simulink model "QueuingSys"  (R2019a)
settings: Solver=VariableStepAuto  StartTime=0.0  StopTime=100  RelTol=1e-3  EnableMultiTasking=on
undefined symbols (not defined in the file or in its folder): m, n
(part 3 of 5)

== system QueuingSys/Distro/MMPPArrivalTime24 ==
  MMPPArrivalTime : TriggerPort  TriggerType=function-call  IsSimulinkFunction=on  FunctionName=MMPPArrivalTime24  VariantControl=Variant
  Constant : Constant  Value=[0.218340938389595 0.112706229136437 0.0913791285356704 0.241717143612315 0.159963629022395 0.101992894543926 0.0739000367596616;0.0360429161526207 0.16434013799063 0.194545292361739 0.260986317842324 0.234076920168349 0.0038388732382826 0.106169542246055;0.140845783996419 0.02142596356304 0.111964255838453 0.214688760468444 0.132405739812884 0.209389328411991 0.169280167908768;0.211603580954734 0.138780880432766 0.228851357631222 0.0929736021625317 0.108365975350849 0.0914026950245187 0.128021908443379;0.196540606477369 0.0424862723550309 0.159462548654797 0.273079768135701 0.0483000474860654 0.264280550522422 0.0158502063686151;0.085539978130616 0.250500965051522 0.0543067416023752 0.49850487643992 0.0486548909117167 0.0235174933555764 0.0389750545082738;0.31220517043653 0.0426377800562429 0.0809275354551289 0.212374582756575 0.0496193007621742 0.129356039135099 0.17287959139825]  SampleTime=-1
  D : Memory  InitialCondition=[0.614629194324132;0.93243288261142]  InheritSampleTime=on
  MMPP : MATLAB Function  TreatAsAtomicUnit=on
  Scope : Scope
  Scope1 : Scope
  T : Memory  InitialCondition=[0 2.63126280993244]  InheritSampleTime=on
  Uniform Random Number : UniformRandomNumber  Minimum=0  Seed=randi(5000)
  X : Memory  InitialCondition=6  InheritSampleTime=on
  t : ArgOut  DisableCoverage=on  ArgumentName=t
  wires:
  MMPP/5(lambda) -> Scope1/1
  D/1 -> MMPP/3("D ")
  MMPP/3(D) -> D/1
  Uniform Random Number/1 -> MMPP/5(rn)
  Constant/1 -> MMPP/4(M)
  MMPP/1(x) -> X/1
  MMPP/4(t) -> Scope/1, t/1
  MMPP/2(T) -> T/1
  T/1 -> MMPP/2("T ")
  X/1 -> MMPP/1("x ")

== system QueuingSys/Distro/MMPPArrivalTime25 ==
  MMPPArrivalTime : TriggerPort  TriggerType=function-call  IsSimulinkFunction=on  FunctionName=MMPPArrivalTime25  VariantControl=Variant
  Constant : Constant  Value=[0.126261776016378 0.256876331205712 0.0743475491381239 0.00987911876596653 0.24041097573006 0.277579906213371 0.0146443429303889;0.215158684388773 0.104699058732068 0.221561488259183 0.114082371425467 0.0931958184132832 0.01898756457891 0.232315014202317;0.14339812125704 0.0963851661286175 0.131725285252208 0.10866184472534 0.104448382274097 0.209437276973192 0.205943923389506;0.11415078083782 0.105394383343145 0.072989249176117 0.0766899189422998 0.184068505318316 0.202592491193927 0.244114671188375;0.280165053993371 0.246511798654403 0.0536757705944194 0.0749268053671436 0.0110419684998257 0.239894108144276 0.0937844947465618;0.127024999749287 0.139114287100631 0.0561443135743664 0.194893192372715 0.202125284585139 0.144969287988396 0.135728634629465;0.0425570718208876 0.00912945422340431 0.179607472937085 0.0477907549956977 0.250445957494757 0.305723190577337 0.16474609795083]  SampleTime=-1
  D : Memory  InitialCondition=[0.84739945723103;0.0464259746177923]  InheritSampleTime=on
  MMPP : MATLAB Function  TreatAsAtomicUnit=on
  Scope : Scope
  Scope1 : Scope
  T : Memory  InitialCondition=[0 0.0425610144779381]  InheritSampleTime=on
  Uniform Random Number : UniformRandomNumber  Minimum=0  Seed=randi(5000)
  X : Memory  InitialCondition=2  InheritSampleTime=on
  t : ArgOut  DisableCoverage=on  ArgumentName=t
  wires:
  MMPP/5(lambda) -> Scope1/1
  D/1 -> MMPP/3("D ")
  MMPP/3(D) -> D/1
  Uniform Random Number/1 -> MMPP/5(rn)
  Constant/1 -> MMPP/4(M)
  MMPP/1(x) -> X/1
  MMPP/4(t) -> Scope/1, t/1
  MMPP/2(T) -> T/1
  T/1 -> MMPP/2("T ")
  X/1 -> MMPP/1("x ")

== system QueuingSys/Distro/MMPPArrivalTime26 ==
  MMPPArrivalTime : TriggerPort  TriggerType=function-call  IsSimulinkFunction=on  FunctionName=MMPPArrivalTime26  VariantControl=Variant
  Constant : Constant  Value=[0.309285239272645 0.083936319045581 0.245188935840708 0.0586916651116355 0.30289784072943;0.249604131350162 0.0262375593681035 0.162014420154344 0.297986672414955 0.264157216712436;0.239496080520532 0.182486674532759 0.050516361065497 0.273833117885605 0.253667765995607;0.323084290176268 0.192126026414458 0.270902867326008 0.0249505358502317 0.188936280233035;0.104368266697699 0.216371091313532 0.330325183296464 0.160531785510462 0.188403673181843]  SampleTime=-1
  D : Memory  InitialCondition=[0.550755647407727;0.0211027090790837]  InheritSampleTime=on
  MMPP : MATLAB Function  TreatAsAtomicUnit=on
  Scope : Scope
  Scope1 : Scope
  T : Memory  InitialCondition=[0 0.0207689449845097]  InheritSampleTime=on
  Uniform Random Number : UniformRandomNumber  Minimum=0  Seed=randi(5000)
  X : Memory  InitialCondition=2  InheritSampleTime=on
  t : ArgOut  DisableCoverage=on  ArgumentName=t
  wires:
  MMPP/5(lambda) -> Scope1/1
  D/1 -> MMPP/3("D ")
  MMPP/3(D) -> D/1
  Uniform Random Number/1 -> MMPP/5(rn)
  Constant/1 -> MMPP/4(M)
  MMPP/1(x) -> X/1
  MMPP/4(t) -> Scope/1, t/1
  MMPP/2(T) -> T/1
  T/1 -> MMPP/2("T ")
  X/1 -> MMPP/1("x ")

== system QueuingSys/Distro/MMPPArrivalTime27 ==
  MMPPArrivalTime : TriggerPort  TriggerType=function-call  IsSimulinkFunction=on  FunctionName=MMPPArrivalTime27  VariantControl=Variant
  Constant : Constant  Value=[0.0196700480561395 0.172600946334506 0.06119529123324 0.251913080143349 0.203718565734216 0.023675877826922 0.267226190671628;0.205861749772008 0.124740430483342 0.0435703487835078 0.259776169203363 0.0251637412405287 0.17177162160965 0.1691159389076;0.0904528149038582 0.0959237307535102 0.0306910128518777 0.237037056690732 0.299086060346327 0.121241544402983 0.125567780050711;0.176070953971679 0.13353863981546 0.0584921398192287 0.131654632433121 0.203364803433442 0.264440012361479 0.0324388181655907;0.00682467460967966 0.136506391709582 0.1695545589303 0.0616100040887452 0.235157640071546 0.244081774115166 0.146264956474981;0.207402505537025 0.0413850634308422 0.182991180389438 0.316311957756415 0.184261630080702 0.0181993774103212 0.0494482853952567;0.145241607470582 0.0447181503479344 0.178772050900297 0.275021549474886 0.104683047120619 0.122449058457546 0.129114536228135]  SampleTime=-1
  D : Memory  InitialCondition=[0.700369541067379;0.242934140773795]  InheritSampleTime=on
  MMPP : MATLAB Function  TreatAsAtomicUnit=on
  Scope : Scope
  Scope1 : Scope
  T : Memory  InitialCondition=[0 0.242371804276988]  InheritSampleTime=on
  Uniform Random Number : UniformRandomNumber  Minimum=0  Seed=randi(5000)
  X : Memory  InitialCondition=7  InheritSampleTime=on
  t : ArgOut  DisableCoverage=on  ArgumentName=t
  wires:
  MMPP/5(lambda) -> Scope1/1
  D/1 -> MMPP/3("D ")
  MMPP/3(D) -> D/1
  Uniform Random Number/1 -> MMPP/5(rn)
  Constant/1 -> MMPP/4(M)
  MMPP/1(x) -> X/1
  MMPP/4(t) -> Scope/1, t/1
  MMPP/2(T) -> T/1
  T/1 -> MMPP/2("T ")
  X/1 -> MMPP/1("x ")

== system QueuingSys/Distro/MMPPArrivalTime28 ==
  MMPPArrivalTime : TriggerPort  TriggerType=function-call  IsSimulinkFunction=on  FunctionName=MMPPArrivalTime28  VariantControl=Variant
  Constant : Constant  Value=[0.1675255939648 0.101797007593022 0.0303730682831272 0.191997428752922 0.177264712643887 0.146387932831963 0.184654255930279;0.0912477542718936 0.210931993970778 0.0843201480116723 0.111897739158023 0.199814913216273 0.20159192162701 0.10019552974435;0.180338394416384 0.0648589650830369 0.154118175392293 0.226715427173359 0.12728298840704 0.0288523571467605 0.217833692381126;0.0172333427169226 0.115598193733394 0.185240713030407 0.185688777825975 0.244050753511532 0.0819293138551697 0.170258905326599;0.157350362929966 0.113879543061761 0.0405457746052219 0.172657753409921 0.145665390816055 0.205649178077014 0.164251997100062;0.0546760945863477 0.153057227941813 0.257667191534973 0.0188514226540526 0.137508337324733 0.175025750837647 0.203213975120434;0.260458682561119 0.122800657363155 0.13819465966866 0.154807542868708 0.145945797704611 0.141207580696075 0.0365850791376733]  SampleTime=-1
  D : Memory  InitialCondition=[0.424539768316478;0.0762116456896338]  InheritSampleTime=on
  MMPP : MATLAB Function  TreatAsAtomicUnit=on
  Scope : Scope
  Scope1 : Scope
  T : Memory  InitialCondition=[0 0.0763721044476675]  InheritSampleTime=on
  Uniform Random Number : UniformRandomNumber  Minimum=0  Seed=randi(5000)
  X : Memory  InitialCondition=7  InheritSampleTime=on
  t : ArgOut  DisableCoverage=on  ArgumentName=t
  wires:
  MMPP/5(lambda) -> Scope1/1
  D/1 -> MMPP/3("D ")
  MMPP/3(D) -> D/1
  Uniform Random Number/1 -> MMPP/5(rn)
  Constant/1 -> MMPP/4(M)
  MMPP/1(x) -> X/1
  MMPP/4(t) -> Scope/1, t/1
  MMPP/2(T) -> T/1
  T/1 -> MMPP/2("T ")
  X/1 -> MMPP/1("x ")

== system QueuingSys/Distro/MMPPArrivalTime29 ==
  MMPPArrivalTime : TriggerPort  TriggerType=function-call  IsSimulinkFunction=on  FunctionName=MMPPArrivalTime29  VariantControl=Variant
  Constant : Constant  Value=[0.470307344262561 0.529692655737439;0.523064675332342 0.476935324667657]  SampleTime=-1
  D : Memory  InitialCondition=[0.726421985150142;0.96965829636015]  InheritSampleTime=on
  MMPP : MATLAB Function  TreatAsAtomicUnit=on
  Scope : Scope
  Scope1 : Scope
  T : Memory  InitialCondition=[0 1.82823247238093]  InheritSampleTime=on
  Uniform Random Number : UniformRandomNumber  Minimum=0  Seed=randi(5000)
  X : Memory  InitialCondition=2  InheritSampleTime=on
  t : ArgOut  DisableCoverage=on  ArgumentName=t
  wires:
  MMPP/5(lambda) -> Scope1/1
  D/1 -> MMPP/3("D ")
  MMPP/3(D) -> D/1
  Uniform Random Number/1 -> MMPP/5(rn)
  Constant/1 -> MMPP/4(M)
  MMPP/1(x) -> X/1
  MMPP/4(t) -> Scope/1, t/1
  MMPP/2(T) -> T/1
  T/1 -> MMPP/2("T ")
  X/1 -> MMPP/1("x ")

== system QueuingSys/Distro/MMPPArrivalTime3 ==
  MMPPArrivalTime : TriggerPort  TriggerType=function-call  IsSimulinkFunction=on  FunctionName=MMPPArrivalTime3  VariantControl=Variant
  Constant : Constant  Value=[0.0853139913388701 0.239102079449207 0.489498373035174 0.186085556176749;0.186029910896899 0.261659421874697 0.139124397204909 0.413186270023495;0.080616426625654 0.578467411552794 0.0755341435246165 0.265382018296936;0.264757301524701 0.239754222585884 0.232748837542538 0.262739638346877]  SampleTime=-1
  D : Memory  InitialCondition=[0.364873259363617;0.592348112171321]  InheritSampleTime=on
  MMPP : MATLAB Function  TreatAsAtomicUnit=on
  Scope : Scope
  Scope1 : Scope
  T : Memory  InitialCondition=[0 0.662543778390372]  InheritSampleTime=on
  Uniform Random Number : UniformRandomNumber  Minimum=0  Seed=randi(5000)
  X : Memory  InitialCondition=2  InheritSampleTime=on
  t : ArgOut  DisableCoverage=on  ArgumentName=t
  wires:
  MMPP/5(lambda) -> Scope1/1
  D/1 -> MMPP/3("D ")
  MMPP/3(D) -> D/1
  Uniform Random Number/1 -> MMPP/5(rn)
  Constant/1 -> MMPP/4(M)
  MMPP/1(x) -> X/1
  MMPP/4(t) -> Scope/1, t/1
  MMPP/2(T) -> T/1
  T/1 -> MMPP/2("T ")
  X/1 -> MMPP/1("x ")

== system QueuingSys/Distro/MMPPArrivalTime30 ==
  MMPPArrivalTime : TriggerPort  TriggerType=function-call  IsSimulinkFunction=on  FunctionName=MMPPArrivalTime30  VariantControl=Variant
  Constant : Constant  Value=[0.206572829547094 0.11219538376502 0.0414783498047576 0.0687166204079749 0.217040951439454 0.0233088998460538 0.330686965189645;0.0588099616266013 0.0794819809807138 0.18046857010927 0.259163205134866 0.1951710016914 0.0924066931854189 0.13449858727173;0.192316426756978 0.190331660158251 0.11812663421486 0.0065555090136078 0.0790712313226722 0.19933171996182 0.214266818571811;0.223545619778498 0.175061907654338 0.150386818941687 0.010317301988908 0.134998537748626 0.173714752944733 0.13197506094321;0.032314357765021 0.23207229786882 0.0750070852278723 0.148072100493113 0.00549085782388581 0.309198074392357 0.197845226428931;0.0617036657326432 0.2510046542784 0.269268599101514 0.0236408275422659 0.0719896733859343 0.318189330143183 0.00420324981605986;0.13091473295952 0.202410050810776 0.0560641524610722 0.212696647631418 0.186442191875069 0.0532754576242078 0.158196766637937]  SampleTime=-1
  D : Memory  InitialCondition=[0.118637485115407;0.596256415905622]  InheritSampleTime=on
  MMPP : MATLAB Function  TreatAsAtomicUnit=on
  Scope : Scope
  Scope1 : Scope
  T : Memory  InitialCondition=[0 0.799837356402608]  InheritSampleTime=on
  Uniform Random Number : UniformRandomNumber  Minimum=0  Seed=randi(5000)
  X : Memory  InitialCondition=3  InheritSampleTime=on
  t : ArgOut  DisableCoverage=on  ArgumentName=t
  wires:
  MMPP/5(lambda) -> Scope1/1
  D/1 -> MMPP/3("D ")
  MMPP/3(D) -> D/1
  Uniform Random Number/1 -> MMPP/5(rn)
  Constant/1 -> MMPP/4(M)
  MMPP/1(x) -> X/1
  MMPP/4(t) -> Scope/1, t/1
  MMPP/2(T) -> T/1
  T/1 -> MMPP/2("T ")
  X/1 -> MMPP/1("x ")

== system QueuingSys/Distro/MMPPArrivalTime31 ==
  MMPPArrivalTime : TriggerPort  TriggerType=function-call  IsSimulinkFunction=on  FunctionName=MMPPArrivalTime31  VariantControl=Variant
  Constant : Constant  Value=[0.551391508708422 0.448608491291578;0.824915716015716 0.175084283984284]  SampleTime=-1
  D : Memory  InitialCondition=[0.92288310288109;0.466638676984603]  InheritSampleTime=on
  MMPP : MATLAB Function  TreatAsAtomicUnit=on
  Scope : Scope
  Scope1 : Scope
  T : Memory  InitialCondition=[0 0.518505871400884]  InheritSampleTime=on
  Uniform Random Number : UniformRandomNumber  Minimum=0  Seed=randi(5000)
  X : Memory  InitialCondition=2  InheritSampleTime=on
  t : ArgOut  DisableCoverage=on  ArgumentName=t
  wires:
  MMPP/5(lambda) -> Scope1/1
  D/1 -> MMPP/3("D ")
  MMPP/3(D) -> D/1
  Uniform Random Number/1 -> MMPP/5(rn)
  Constant/1 -> MMPP/4(M)
  MMPP/1(x) -> X/1
  MMPP/4(t) -> Scope/1, t/1
  MMPP/2(T) -> T/1
  T/1 -> MMPP/2("T ")
  X/1 -> MMPP/1("x ")

== system QueuingSys/Distro/MMPPArrivalTime32 ==
  MMPPArrivalTime : TriggerPort  TriggerType=function-call  IsSimulinkFunction=on  FunctionName=MMPPArrivalTime32  VariantControl=Variant
  Constant : Constant  Value=[0.344522048946834 0.136306917950239 0.243903798161791 0.275267234941136;0.06886895570874 0.352562593749696 0.352121845604469 0.226446604937095;0.30079890177196 0.413635172818291 0.147841511174284 0.137724414235466;0.376216524611495 0.161598610656973 0.00958590106540561 0.452598963666126]  SampleTime=-1
  D : Memory  InitialCondition=[0.488629533539644;0.697627838276884]  InheritSampleTime=on
  MMPP : MATLAB Function  TreatAsAtomicUnit=on
  Scope : Scope
  Scope1 : Scope
  T : Memory  InitialCondition=[0 0.654744571333629]  InheritSampleTime=on
  Uniform Random Number : UniformRandomNumber  Minimum=0  Seed=randi(5000)
  X : Memory  InitialCondition=4  InheritSampleTime=on
  t : ArgOut  DisableCoverage=on  ArgumentName=t
  wires:
  MMPP/5(lambda) -> Scope1/1
  D/1 -> MMPP/3("D ")
  MMPP/3(D) -> D/1
  Uniform Random Number/1 -> MMPP/5(rn)
  Constant/1 -> MMPP/4(M)
  MMPP/1(x) -> X/1
  MMPP/4(t) -> Scope/1, t/1
  MMPP/2(T) -> T/1
  T/1 -> MMPP/2("T ")
  X/1 -> MMPP/1("x ")

== system QueuingSys/Distro/MMPPArrivalTime33 ==
  MMPPArrivalTime : TriggerPort  TriggerType=function-call  IsSimulinkFunction=on  FunctionName=MMPPArrivalTime33  VariantControl=Variant
  Constant : Constant  Value=[0.171570956465584 0.260364817442339 0.320191290579991 0.1239189983333 0.123953937178787;0.179651339948253 0.325383097134665 0.272114117246603 0.0546771683346933 0.168174277335786;0.232175063373843 0.0522707652618958 0.22964458887778 0.278757495659698 0.207152086826784;0.10404887259382 0.143469750206921 0.301159993610954 0.341816203786128 0.109505179802177;0.131507997957578 0.0534805913519804 0.316881075206008 0.419095285263278 0.0790350502211546]  SampleTime=-1
  D : Memory  InitialCondition=[0.347441299611992;0.139538463016827]  InheritSampleTime=on
  MMPP : MATLAB Function  TreatAsAtomicUnit=on
  Scope : Scope
  Scope1 : Scope
  T : Memory  InitialCondition=[0 0.101385720601707]  InheritSampleTime=on
  Uniform Random Number : UniformRandomNumber  Minimum=0  Seed=randi(5000)
  X : Memory  InitialCondition=2  InheritSampleTime=on
  t : ArgOut  DisableCoverage=on  ArgumentName=t
  wires:
  MMPP/5(lambda) -> Scope1/1
  D/1 -> MMPP/3("D ")
  MMPP/3(D) -> D/1
  Uniform Random Number/1 -> MMPP/5(rn)
  Constant/1 -> MMPP/4(M)
  MMPP/1(x) -> X/1
  MMPP/4(t) -> Scope/1, t/1
  MMPP/2(T) -> T/1
  T/1 -> MMPP/2("T ")
  X/1 -> MMPP/1("x ")

== system QueuingSys/Distro/MMPPArrivalTime34 ==
  MMPPArrivalTime : TriggerPort  TriggerType=function-call  IsSimulinkFunction=on  FunctionName=MMPPArrivalTime34  VariantControl=Variant
  Constant : Constant  Value=[0.279863661105788 0.018954509277061 0.701181829617151;0.102024833223184 0.172747068074691 0.725228098702125;0.384615776864446 0.575978320906199 0.0394059022293549]  SampleTime=-1
  D : Memory  InitialCondition=[0.423405961364762;0.537076428867559]  InheritSampleTime=on
  MMPP : MATLAB Function  TreatAsAtomicUnit=on
  Scope : Scope
  Scope1 : Scope
  T : Memory  InitialCondition=[0 0.554644191706879]  InheritSampleTime=on
  Uniform Random Number : UniformRandomNumber  Minimum=0  Seed=randi(5000)
  X : Memory  InitialCondition=1  InheritSampleTime=on
  t : ArgOut  DisableCoverage=on  ArgumentName=t
  wires:
  MMPP/5(lambda) -> Scope1/1
  D/1 -> MMPP/3("D ")
  MMPP/3(D) -> D/1
  Uniform Random Number/1 -> MMPP/5(rn)
  Constant/1 -> MMPP/4(M)
  MMPP/1(x) -> X/1
  MMPP/4(t) -> Scope/1, t/1
  MMPP/2(T) -> T/1
  T/1 -> MMPP/2("T ")
  X/1 -> MMPP/1("x ")

== system QueuingSys/Distro/MMPPArrivalTime35 ==
  MMPPArrivalTime : TriggerPort  TriggerType=function-call  IsSimulinkFunction=on  FunctionName=MMPPArrivalTime35  VariantControl=Variant
  Constant : Constant  Value=[0.188780303843234 0.0823697536250097 0.299442601204683 0.146155756238697 0.283251585088376;0.194799765979573 0.191388575346313 0.213506643310004 0.133027575958572 0.267277439405539;0.16877861121083 0.164421712552048 0.17530282851964 0.169585093051173 0.321911754666309;0.0315952166008945 0.440650528842051 0.356378180470412 0.151542346675446 0.0198337274111962;0.265589533235786 0.370378088201544 0.0329951268661805 0.0974786689921767 0.233558582704313]  SampleTime=-1
  D : Memory  InitialCondition=[0.246188510868016;0.398386263151892]  InheritSampleTime=on
  MMPP : MATLAB Function  TreatAsAtomicUnit=on
  Scope : Scope
  Scope1 : Scope
  T : Memory  InitialCondition=[0 0.419061350834402]  InheritSampleTime=on
  Uniform Random Number : UniformRandomNumber  Minimum=0  Seed=randi(5000)
  X : Memory  InitialCondition=3  InheritSampleTime=on
  t : ArgOut  DisableCoverage=on  ArgumentName=t
  wires:
  MMPP/5(lambda) -> Scope1/1
  D/1 -> MMPP/3("D ")
  MMPP/3(D) -> D/1
  Uniform Random Number/1 -> MMPP/5(rn)
  Constant/1 -> MMPP/4(M)
  MMPP/1(x) -> X/1
  MMPP/4(t) -> Scope/1, t/1
  MMPP/2(T) -> T/1
  T/1 -> MMPP/2("T ")
  X/1 -> MMPP/1("x ")

== system QueuingSys/Distro/MMPPArrivalTime36 ==
  MMPPArrivalTime : TriggerPort  TriggerType=function-call  IsSimulinkFunction=on  FunctionName=MMPPArrivalTime36  VariantControl=Variant
  Constant : Constant  Value=[0.0721368925951376 0.0990877542742027 0.15766762160974 0.173717021931805 0.232520566458114 0.215181743087032 0.0496884000439679;0.104345427832741 0.304945840868097 0.0957926029195893 0.00143421589660746 0.241314256300479 0.00825440376825492 0.243913252414231;0.12349090907902 0.00664393290749279 0.245300465357095 0.0195344479846606 0.147185959478393 0.114720921424828 0.343123363768511;0.0112228226668296 0.212190536597801 0.0609153022626635 0.0522158319742919 0.273310886164233 0.275703567304479 0.114441053029702;0.251806028010796 0.15155975988215 0.0742686826241297 0.0919408199460609 0.0677486819667469 0.324470433888815 0.0382055936813014;0.240353492122863 0.0821997319260256 0.101915103790219 0.153099504996242 0.217093033969166 0.0556167959155748 0.14972233727991;0.203394006302543 0.197611226075048 0.00526531609215853 0.0598232661159766 0.203224493959019 0.165643705328875 0.165037986126379]  SampleTime=-1
  D : Memory  InitialCondition=[0.865261678105272;0.48778428565265]  InheritSampleTime=on
  MMPP : MATLAB Function  TreatAsAtomicUnit=on
  Scope : Scope
  Scope1 : Scope
  T : Memory  InitialCondition=[0 0.620749164508373]  InheritSampleTime=on
  Uniform Random Number : UniformRandomNumber  Minimum=0  Seed=randi(5000)
  X : Memory  InitialCondition=1  InheritSampleTime=on
  t : ArgOut  DisableCoverage=on  ArgumentName=t
  wires:
  MMPP/5(lambda) -> Scope1/1
  D/1 -> MMPP/3("D ")
  MMPP/3(D) -> D/1
  Uniform Random Number/1 -> MMPP/5(rn)
  Constant/1 -> MMPP/4(M)
  MMPP/1(x) -> X/1
  MMPP/4(t) -> Scope/1, t/1
  MMPP/2(T) -> T/1
  T/1 -> MMPP/2("T ")
  X/1 -> MMPP/1("x ")

== system QueuingSys/Distro/MMPPArrivalTime37 ==
  MMPPArrivalTime : TriggerPort  TriggerType=function-call  IsSimulinkFunction=on  FunctionName=MMPPArrivalTime37  VariantControl=Variant
  Constant : Constant  Value=[0.441689750469483 0.131529499484869 0.426780750045648;0.287185036754023 0.0687395784305002 0.644075384815477;0.412359757912282 0.228704386513075 0.358935855574643]  SampleTime=-1
  D : Memory  InitialCondition=[0.206323180349956;0.156967245259197]  InheritSampleTime=on
  MMPP : MATLAB Function  TreatAsAtomicUnit=on
  Scope : Scope
  Scope1 : Scope
  T : Memory  InitialCondition=[0 0.159012220401242]  InheritSampleTime=on
  Uniform Random Number : UniformRandomNumber  Minimum=0  Seed=randi(5000)
  X : Memory  InitialCondition=2  InheritSampleTime=on
  t : ArgOut  DisableCoverage=on  ArgumentName=t
  wires:
  MMPP/5(lambda) -> Scope1/1
  D/1 -> MMPP/3("D ")
  MMPP/3(D) -> D/1
  Uniform Random Number/1 -> MMPP/5(rn)
  Constant/1 -> MMPP/4(M)
  MMPP/1(x) -> X/1
  MMPP/4(t) -> Scope/1, t/1
  MMPP/2(T) -> T/1
  T/1 -> MMPP/2("T ")
  X/1 -> MMPP/1("x ")

== system QueuingSys/Distro/MMPPArrivalTime38 ==
  MMPPArrivalTime : TriggerPort  TriggerType=function-call  IsSimulinkFunction=on  FunctionName=MMPPArrivalTime38  VariantControl=Variant
  Constant : Constant  Value=[0.287926085776875 0.326808914343824 0.140791705619385 0.244473294259917;0.0921151970194848 0.566376965300379 0.244906087745248 0.0966017499348885;0.062348026383559 0.393080925446152 0.351838246969326 0.192732801200964;0.184965879275065 0.287580878998744 0.309163942419966 0.218289299306224]  SampleTime=-1
  D : Memory  InitialCondition=[0.828422805979749;0.99837009190541]  InheritSampleTime=on
  MMPP : MATLAB Function  TreatAsAtomicUnit=on
  Scope : Scope
  Scope1 : Scope
  T : Memory  InitialCondition=[0 4.16070043901108]  InheritSampleTime=on
  Uniform Random Number : UniformRandomNumber  Minimum=0  Seed=randi(5000)
  X : Memory  InitialCondition=3  InheritSampleTime=on
  t : ArgOut  DisableCoverage=on  ArgumentName=t
  wires:
  MMPP/5(lambda) -> Scope1/1
  D/1 -> MMPP/3("D ")
  MMPP/3(D) -> D/1
  Uniform Random Number/1 -> MMPP/5(rn)
  Constant/1 -> MMPP/4(M)
  MMPP/1(x) -> X/1
  MMPP/4(t) -> Scope/1, t/1
  MMPP/2(T) -> T/1
  T/1 -> MMPP/2("T ")
  X/1 -> MMPP/1("x ")

== system QueuingSys/Distro/MMPPArrivalTime39 ==
  MMPPArrivalTime : TriggerPort  TriggerType=function-call  IsSimulinkFunction=on  FunctionName=MMPPArrivalTime39  VariantControl=Variant
  Constant : Constant  Value=[0.203369723433177 0.0981529295965351 0.27974031168011 0.418737035290178;0.118401652360432 0.343942875686384 0.483441151549918 0.0542143204032651;0.57842810044429 0.0186327882062443 0.0993934778872626 0.303545633462203;0.181636059897378 0.250261790687725 0.21359752945179 0.354504619963107]  SampleTime=-1
  D : Memory  InitialCondition=[0.700194935136202;0.830731114447627]  InheritSampleTime=on
  MMPP : MATLAB Function  TreatAsAtomicUnit=on
  Scope : Scope
  Scope1 : Scope
  T : Memory  InitialCondition=[0 1.41502790389446]  InheritSampleTime=on
  Uniform Random Number : UniformRandomNumber  Minimum=0  Seed=randi(5000)
  X : Memory  InitialCondition=1  InheritSampleTime=on
  t : ArgOut  DisableCoverage=on  ArgumentName=t
  wires:
  MMPP/5(lambda) -> Scope1/1
  D/1 -> MMPP/3("D ")
  MMPP/3(D) -> D/1
  Uniform Random Number/1 -> MMPP/5(rn)
  Constant/1 -> MMPP/4(M)
  MMPP/1(x) -> X/1
  MMPP/4(t) -> Scope/1, t/1
  MMPP/2(T) -> T/1
  T/1 -> MMPP/2("T ")
  X/1 -> MMPP/1("x ")

== system QueuingSys/Distro/MMPPArrivalTime4 ==
  MMPPArrivalTime : TriggerPort  TriggerType=function-call  IsSimulinkFunction=on  FunctionName=MMPPArrivalTime4  VariantControl=Variant
  Constant : Constant  Value=[0.0222433821916003 0.188004075907925 0.0437472879804383 0.12935035710123 0.178735535005156 0.182042759176272 0.0734492807049325 0.182427321932446;0.114137403815038 0.118952869883947 0.173447243215089 0.0309547927779365 0.09532864645341 0.142509570506958 0.0965657578792342 0.228103715468389;0.149811893306025 0.0250072529977261 0.082539304657149 0.106939407254426 0.184206355648754 0.186347503583938 0.0910378188644563 0.174110463687526;0.199110919696702 0.0774059631971286 0.114567260154314 0.166430806338449 0.0700866595008907 0.191021231764798 0.154458031307493 0.0269191280402247;0.136518653768493 0.189298811903415 0.0490924625299025 0.0850191815014507 0.113079738549474 0.0120577465523648 0.226651515000193 0.188281890194708;0.010143876364335 0.212656924819349 0.0912173901823647 0.115440804587796 0.0551317551617981 0.226660862641394 0.14582232951616 0.142926056726803;0.129649913543163 0.154270484050175 0.0757750971600601 0.0262850321230364 0.171745147765562 0.140824816060237 0.212889797246578 0.088559712051188;0.0675108333403751 0.235392828283239 0.0864519004234807 0.139572546540988 0.06630522993186 0.0176149303934803 0.183129017966379 0.204022713120198]  SampleTime=-1
  D : Memory  InitialCondition=[0.0962059280401967;0.948102236245469]  InheritSampleTime=on
  MMPP : MATLAB Function  TreatAsAtomicUnit=on
  Scope : Scope
  Scope1 : Scope
  T : Memory  InitialCondition=[0 2.89267298537551]  InheritSampleTime=on
  Uniform Random Number : UniformRandomNumber  Minimum=0  Seed=randi(5000)
  X : Memory  InitialCondition=1  InheritSampleTime=on
  t : ArgOut  DisableCoverage=on  ArgumentName=t
  wires:
  MMPP/5(lambda) -> Scope1/1
  D/1 -> MMPP/3("D ")
  MMPP/3(D) -> D/1
  Uniform Random Number/1 -> MMPP/5(rn)
  Constant/1 -> MMPP/4(M)
  MMPP/1(x) -> X/1
  MMPP/4(t) -> Scope/1, t/1
  MMPP/2(T) -> T/1
  T/1 -> MMPP/2("T ")
  X/1 -> MMPP/1("x ")

== system QueuingSys/Distro/MMPPArrivalTime40 ==
  MMPPArrivalTime : TriggerPort  TriggerType=function-call  IsSimulinkFunction=on  FunctionName=MMPPArrivalTime40  VariantControl=Variant
  Constant : Constant  Value=[0.307578865869595 0.132038010112806 0.121090750876633 0.221383495684156 0.21790887745681;0.0744758422654912 0.243685342092243 0.270264233257038 0.242878524139999 0.16869605824523;0.0720937486394534 0.228376662965373 0.214644675250443 0.235434871797632 0.249450041347098;0.213128802454875 0.258371791749583 0.259796810506448 0.00747698392181957 0.261225611367275;0.231301535709266 0.178744002603726 0.184654760537249 0.173233407727554 0.232066293422205]  SampleTime=-1
  D : Memory  InitialCondition=[0.277363250387578;0.316407242248477]  InheritSampleTime=on
  MMPP : MATLAB Function  TreatAsAtomicUnit=on
  Scope : Scope
  Scope1 : Scope
  T : Memory  InitialCondition=[0 0.287696742729591]  InheritSampleTime=on
  Uniform Random Number : UniformRandomNumber  Minimum=0  Seed=randi(5000)
  X : Memory  InitialCondition=2  InheritSampleTime=on
  t : ArgOut  DisableCoverage=on  ArgumentName=t
  wires:
  MMPP/5(lambda) -> Scope1/1
  D/1 -> MMPP/3("D ")
  MMPP/3(D) -> D/1
  Uniform Random Number/1 -> MMPP/5(rn)
  Constant/1 -> MMPP/4(M)
  MMPP/1(x) -> X/1
  MMPP/4(t) -> Scope/1, t/1
  MMPP/2(T) -> T/1
  T/1 -> MMPP/2("T ")
  X/1 -> MMPP/1("x ")

== system QueuingSys/Distro/MMPPArrivalTime41 ==
  MMPPArrivalTime : TriggerPort  TriggerType=function-call  IsSimulinkFunction=on  FunctionName=MMPPArrivalTime41  VariantControl=Variant
  Constant : Constant  Value=[0.410876353322907 0.0584260983388013 0.337581915528107 0.193115632810185;0.335369397531136 0.236701922750816 0.19284870942629 0.235079970291758;0.202496633153807 0.0925488926150038 0.323559931884597 0.381394542346592;0.232535225417897 0.0796771501394147 0.072060247438763 0.615727377003925]  SampleTime=-1
  D : Memory  InitialCondition=[0.372362436968764;0.102235461961869]  InheritSampleTime=on
  MMPP : MATLAB Function  TreatAsAtomicUnit=on
  Scope : Scope
  Scope1 : Scope
  T : Memory  InitialCondition=[0 0.0823197528598087]  InheritSampleTime=on
  Uniform Random Number : UniformRandomNumber  Minimum=0  Seed=randi(5000)
  X : Memory  InitialCondition=2  InheritSampleTime=on
  t : ArgOut  DisableCoverage=on  ArgumentName=t
  wires:
  MMPP/5(lambda) -> Scope1/1
  D/1 -> MMPP/3("D ")
  MMPP/3(D) -> D/1
  Uniform Random Number/1 -> MMPP/5(rn)
  Constant/1 -> MMPP/4(M)
  MMPP/1(x) -> X/1
  MMPP/4(t) -> Scope/1, t/1
  MMPP/2(T) -> T/1
  T/1 -> MMPP/2("T ")
  X/1 -> MMPP/1("x ")

== system QueuingSys/Distro/MMPPArrivalTime42 ==
  MMPPArrivalTime : TriggerPort  TriggerType=function-call  IsSimulinkFunction=on  FunctionName=MMPPArrivalTime42  VariantControl=Variant
  Constant : Constant  Value=[0.19484043500199 0.284944522797008 0.0475706332073199 0.109134773917783 0.239436419068973 0.124073216006926;0.126050594916668 0.261824844654131 0.0248899095858524 0.311802037053651 0.215696750369367 0.0597358634203302;0.0495412974773776 0.210291104549826 0.16361300927134 0.279547564424455 0.191625022747464 0.105382001529537;0.154861130114456 0.239858888632055 0.0256755968521409 0.261586392968357 0.0592600681071114 0.25875792332588;0.244180818964456 0.22217501763753 0.1126239642831 0.0654110364937203 0.137653601903044 0.217955560718149;0.400637514695211 0.318208115296665 0.130290915360653 0.0202519126212345 0.0232855982319286 0.107325943794308]  SampleTime=-1
  D : Memory  InitialCondition=[0.733514334816772;0.782224136821224]  InheritSampleTime=on
  MMPP : MATLAB Function  TreatAsAtomicUnit=on
  Scope : Scope
  Scope1 : Scope
  T : Memory  InitialCondition=[0 1.2748954024409]  InheritSampleTime=on
  Uniform Random Number : UniformRandomNumber  Minimum=0  Seed=randi(5000)
  X : Memory  InitialCondition=3  InheritSampleTime=on
  t : ArgOut  DisableCoverage=on  ArgumentName=t
  wires:
  MMPP/5(lambda) -> Scope1/1
  D/1 -> MMPP/3("D ")
  MMPP/3(D) -> D/1
  Uniform Random Number/1 -> MMPP/5(rn)
  Constant/1 -> MMPP/4(M)
  MMPP/1(x) -> X/1
  MMPP/4(t) -> Scope/1, t/1
  MMPP/2(T) -> T/1
  T/1 -> MMPP/2("T ")
  X/1 -> MMPP/1("x ")

== system QueuingSys/Distro/MMPPArrivalTime43 ==
  MMPPArrivalTime : TriggerPort  TriggerType=function-call  IsSimulinkFunction=on  FunctionName=MMPPArrivalTime43  VariantControl=Variant
  Constant : Constant  Value=[0.666230645010512 0.333769354989488;0.648952377526222 0.351047622473778]  SampleTime=-1
  D : Memory  InitialCondition=[0.695748329396229;0.694899405806817]  InheritSampleTime=on
  MMPP : MATLAB Function  TreatAsAtomicUnit=on
  Scope : Scope
  Scope1 : Scope
  T : Memory  InitialCondition=[0 0.770380283788956]  InheritSampleTime=on
  Uniform Random Number : UniformRandomNumber  Minimum=0  Seed=randi(5000)
  X : Memory  InitialCondition=2  InheritSampleTime=on
  t : ArgOut  DisableCoverage=on  ArgumentName=t
  wires:
  MMPP/5(lambda) -> Scope1/1
  D/1 -> MMPP/3("D ")
  MMPP/3(D) -> D/1
  Uniform Random Number/1 -> MMPP/5(rn)
  Constant/1 -> MMPP/4(M)
  MMPP/1(x) -> X/1
  MMPP/4(t) -> Scope/1, t/1
  MMPP/2(T) -> T/1
  T/1 -> MMPP/2("T ")
  X/1 -> MMPP/1("x ")

== system QueuingSys/Distro/MMPPArrivalTime44 ==
  MMPPArrivalTime : TriggerPort  TriggerType=function-call  IsSimulinkFunction=on  FunctionName=MMPPArrivalTime44  VariantControl=Variant
  Constant : Constant  Value=[0.15203561034492 0.187503181484866 0.217099640527759 0.261940593187943 0.111892281007731 0.000650429792438285 0.0688782636543432;0.0629211458311256 0.261964703771416 0.195749518075014 0.0286599345113848 0.245131323254798 0.102903898094534 0.102669476461728;0.200682855577231 0.138658530834025 0.143251811474266 0.0529877333897891 0.138171464438406 0.141119359774842 0.18512824451144;0.191890770111757 0.437124293431787 0.0315258938631034 0.226728507658625 0.0913806175234772 0.0203987673434622 0.000951150067788178;0.136393955971383 0.0241916835568405 0.18780202494869 0.163005280150987 0.179085451974293 0.120692281793856 0.188829321603951;0.148892943828847 0.235368435604696 0.170914905612149 0.170876773227261 0.0196435783696241 0.0970585690252984 0.157244794332124;0.160582990055915 0.0115380956607863 0.0970534935676632 0.121345310071338 0.21807668732859 0.162514380533904 0.228889042781804]  SampleTime=-1
  D : Memory  InitialCondition=[0.390100290285044;0.951080809713353]  InheritSampleTime=on
  MMPP : MATLAB Function  TreatAsAtomicUnit=on
  Scope : Scope
  Scope1 : Scope
  T : Memory  InitialCondition=[0 2.58531092805497]  InheritSampleTime=on
  Uniform Random Number : UniformRandomNumber  Minimum=0  Seed=randi(5000)
  X : Memory  InitialCondition=3  InheritSampleTime=on
  t : ArgOut  DisableCoverage=on  ArgumentName=t
  wires:
  MMPP/5(lambda) -> Scope1/1
  D/1 -> MMPP/3("D ")
  MMPP/3(D) -> D/1
  Uniform Random Number/1 -> MMPP/5(rn)
  Constant/1 -> MMPP/4(M)
  MMPP/1(x) -> X/1
  MMPP/4(t) -> Scope/1, t/1
  MMPP/2(T) -> T/1
  T/1 -> MMPP/2("T ")
  X/1 -> MMPP/1("x ")

== system QueuingSys/Distro/MMPPArrivalTime45 ==
  MMPPArrivalTime : TriggerPort  TriggerType=function-call  IsSimulinkFunction=on  FunctionName=MMPPArrivalTime45  VariantControl=Variant
  Constant : Constant  Value=[0.208332003253337 0.0984433340257894 0.0275476333176013 0.208455019743088 0.187769647373873 0.138168787674138 0.131283574612174;0.119543919326924 0.030488950877573 0.176370764184541 0.179747392102269 0.16774180681458 0.183564418114314 0.142542748579799;0.0172780841585348 0.295546396625372 0.258578259992568 0.227118085955286 0.132218391124284 0.0520412705413815 0.0172195116025731;0.351815240726735 0.0479964117693768 0.0570504295879172 0.233496406215703 0.0264590985001854 0.265698725665895 0.0174836875341881;0.0156438106290037 0.203879845806784 0.106041292079691 0.227281290089628 0.244940838010454 0.0449931946230161 0.157219728761424;0.078251026730738 0.201058916592686 0.145343733254437 0.118734781147526 0.192447945467668 0.0249161137048323 0.239247483102113;0.0964831958453108 0.0788638465842378 0.189772507959354 0.231147832892259 0.192992728438768 0.163089502009768 0.0476503862703027]  SampleTime=-1
  D : Memory  InitialCondition=[0.573696348603338;0.604938867660859]  InheritSampleTime=on
  MMPP : MATLAB Function  TreatAsAtomicUnit=on
  Scope : Scope
  Scope1 : Scope
  T : Memory  InitialCondition=[0 0.71186320163139]  InheritSampleTime=on
  Uniform Random Number : UniformRandomNumber  Minimum=0  Seed=randi(5000)
  X : Memory  InitialCondition=4  InheritSampleTime=on
  t : ArgOut  DisableCoverage=on  ArgumentName=t
  wires:
  MMPP/5(lambda) -> Scope1/1
  D/1 -> MMPP/3("D ")
  MMPP/3(D) -> D/1
  Uniform Random Number/1 -> MMPP/5(rn)
  Constant/1 -> MMPP/4(M)
  MMPP/1(x) -> X/1
  MMPP/4(t) -> Scope/1, t/1
  MMPP/2(T) -> T/1
  T/1 -> MMPP/2("T ")
  X/1 -> MMPP/1("x ")

== system QueuingSys/Distro/MMPPArrivalTime46 ==
  MMPPArrivalTime : TriggerPort  TriggerType=function-call  IsSimulinkFunction=on  FunctionName=MMPPArrivalTime46  VariantControl=Variant
  Constant : Constant  Value=[0.526814867969532 0.473185132030468;0.0348504552695229 0.965149544730477]  SampleTime=-1
  D : Memory  InitialCondition=[0.370318725663683;0.075636685022303]  InheritSampleTime=on
  MMPP : MATLAB Function  TreatAsAtomicUnit=on
  Scope : Scope
  Scope1 : Scope
  T : Memory  InitialCondition=[0 0.0372160516095348]  InheritSampleTime=on
  Uniform Random Number : UniformRandomNumber  Minimum=0  Seed=randi(5000)
  X : Memory  InitialCondition=1  InheritSampleTime=on
  t : ArgOut  DisableCoverage=on  ArgumentName=t
  wires:
  MMPP/5(lambda) -> Scope1/1
  D/1 -> MMPP/3("D ")
  MMPP/3(D) -> D/1
  Uniform Random Number/1 -> MMPP/5(rn)
  Constant/1 -> MMPP/4(M)
  MMPP/1(x) -> X/1
  MMPP/4(t) -> Scope/1, t/1
  MMPP/2(T) -> T/1
  T/1 -> MMPP/2("T ")
  X/1 -> MMPP/1("x ")

== system QueuingSys/Distro/MMPPArrivalTime47 ==
  MMPPArrivalTime : TriggerPort  TriggerType=function-call  IsSimulinkFunction=on  FunctionName=MMPPArrivalTime47  VariantControl=Variant
  Constant : Constant  Value=[0.357649279094256 0.383062766136625 0.259287954769119;0.18487698933807 0.307582643317699 0.507540367344231;0.302376740201481 0.447645097081492 0.249978162717027]  SampleTime=-1
  D : Memory  InitialCondition=[0.929496207556362;0.418572454279479]  InheritSampleTime=on
  MMPP : MATLAB Function  TreatAsAtomicUnit=on
  Scope : Scope
  Scope1 : Scope
  T : Memory  InitialCondition=[0 0.348326827652435]  InheritSampleTime=on
  Uniform Random Number : UniformRandomNumber  Minimum=0  Seed=randi(5000)
  X : Memory  InitialCondition=1  InheritSampleTime=on
  t : ArgOut  DisableCoverage=on  ArgumentName=t
  wires:
  MMPP/5(lambda) -> Scope1/1
  D/1 -> MMPP/3("D ")
  MMPP/3(D) -> D/1
  Uniform Random Number/1 -> MMPP/5(rn)
  Constant/1 -> MMPP/4(M)
  MMPP/1(x) -> X/1
  MMPP/4(t) -> Scope/1, t/1
  MMPP/2(T) -> T/1
  T/1 -> MMPP/2("T ")
  X/1 -> MMPP/1("x ")

== system QueuingSys/Distro/MMPPArrivalTime48 ==
  MMPPArrivalTime : TriggerPort  TriggerType=function-call  IsSimulinkFunction=on  FunctionName=MMPPArrivalTime48  VariantControl=Variant
  Constant : Constant  Value=[0.0989361828816905 0.178257670888535 0.142181889481987 0.322312499159869 0.258311757587918;0.225531062681923 0.243602356421045 0.15415192697207 0.165161105172416 0.211553548752546;0.205474509467409 0.190905839449352 0.183780085282627 0.165890917526993 0.253948648273619;0.346999335019431 0.174541386602823 0.0398510890529728 0.0705196289089337 0.36808856041584;0.167273984423134 0.205900307853727 0.113969465774524 0.108299928616902 0.404556313331712]  SampleTime=-1
  D : Memory  InitialCondition=[0.529638235684598;0.288370830577306]  InheritSampleTime=on
  MMPP : MATLAB Function  TreatAsAtomicUnit=on
  Scope : Scope
  Scope1 : Scope
  T : Memory  InitialCondition=[0 0.202568949428109]  InheritSampleTime=on
  Uniform Random Number : UniformRandomNumber  Minimum=0  Seed=randi(5000)
  X : Memory  InitialCondition=5  InheritSampleTime=on
  t : ArgOut  DisableCoverage=on  ArgumentName=t
  wires:
  MMPP/5(lambda) -> Scope1/1
  D/1 -> MMPP/3("D ")
  MMPP/3(D) -> D/1
  Uniform Random Number/1 -> MMPP/5(rn)
  Constant/1 -> MMPP/4(M)
  MMPP/1(x) -> X/1
  MMPP/4(t) -> Scope/1, t/1
  MMPP/2(T) -> T/1
  T/1 -> MMPP/2("T ")
  X/1 -> MMPP/1("x ")

== system QueuingSys/Distro/MMPPArrivalTime49 ==
  MMPPArrivalTime : TriggerPort  TriggerType=function-call  IsSimulinkFunction=on  FunctionName=MMPPArrivalTime49  VariantControl=Variant
  Constant : Constant  Value=[0.0169370390093233 0.573595038383496 0.409467922607181;0.279966128744602 0.301329869356476 0.418704001898922;0.00372472863765805 0.113664329342455 0.882610942019887]  SampleTime=-1
  D : Memory  InitialCondition=[0.523322004017897;0.392486014299919]  InheritSampleTime=on
  MMPP : MATLAB Function  TreatAsAtomicUnit=on
  Scope : Scope
  Scope1 : Scope
  T : Memory  InitialCondition=[0 0.348203277213396]  InheritSampleTime=on
  Uniform Random Number : UniformRandomNumber  Minimum=0  Seed=randi(5000)
  X : Memory  InitialCondition=2  InheritSampleTime=on
  t : ArgOut  DisableCoverage=on  ArgumentName=t
  wires:
  MMPP/5(lambda) -> Scope1/1
  D/1 -> MMPP/3("D ")
  MMPP/3(D) -> D/1
  Uniform Random Number/1 -> MMPP/5(rn)
  Constant/1 -> MMPP/4(M)
  MMPP/1(x) -> X/1
  MMPP/4(t) -> Scope/1, t/1
  MMPP/2(T) -> T/1
  T/1 -> MMPP/2("T ")
  X/1 -> MMPP/1("x ")

== system QueuingSys/Distro/MMPPArrivalTime5 ==
  MMPPArrivalTime : TriggerPort  TriggerType=function-call  IsSimulinkFunction=on  FunctionName=MMPPArrivalTime5  VariantControl=Variant
  Constant : Constant  Value=[0.190433648778553 0.311290627479789 0.290257210078387 0.208018513663271;0.0545287179524431 0.45550681599807 0.213399191698696 0.276565274350791;0.32709725875407 0.0520384576738759 0.247760062991669 0.373104220580386;0.321656492085376 0.499520802863322 0.0497368589714937 0.129085846079808]  SampleTime=-1
  D : Memory  InitialCondition=[0.193494994981051;0.53092770419017]  InheritSampleTime=on
  MMPP : MATLAB Function  TreatAsAtomicUnit=on
  Scope : Scope
  Scope1 : Scope
  T : Memory  InitialCondition=[0 0.659280598034344]  InheritSampleTime=on
  Uniform Random Number : UniformRandomNumber  Minimum=0  Seed=randi(5000)
  X : Memory  InitialCondition=4  InheritSampleTime=on
  t : ArgOut  DisableCoverage=on  ArgumentName=t
  wires:
  MMPP/5(lambda) -> Scope1/1
  D/1 -> MMPP/3("D ")
  MMPP/3(D) -> D/1
  Uniform Random Number/1 -> MMPP/5(rn)
  Constant/1 -> MMPP/4(M)
  MMPP/1(x) -> X/1
  MMPP/4(t) -> Scope/1, t/1
  MMPP/2(T) -> T/1
  T/1 -> MMPP/2("T ")
  X/1 -> MMPP/1("x ")

== system QueuingSys/Distro/MMPPArrivalTime50 ==
  MMPPArrivalTime : TriggerPort  TriggerType=function-call  IsSimulinkFunction=on  FunctionName=MMPPArrivalTime50  VariantControl=Variant
  Constant : Constant  Value=[0.710640218684484 0.289359781315516;0.438035940675537 0.561964059324463]  SampleTime=-1
  D : Memory  InitialCondition=[0.737876332989012;0.13841777189992]  InheritSampleTime=on
  MMPP : MATLAB Function  TreatAsAtomicUnit=on
  Scope : Scope
  Scope1 : Scope
  T : Memory  InitialCondition=[0 0.065260688243774]  InheritSampleTime=on
  Uniform Random Number : UniformRandomNumber  Minimum=0  Seed=randi(5000)
  X : Memory  InitialCondition=2  InheritSampleTime=on
  t : ArgOut  DisableCoverage=on  ArgumentName=t
  wires:
  MMPP/5(lambda) -> Scope1/1
  D/1 -> MMPP/3("D ")
  MMPP/3(D) -> D/1
  Uniform Random Number/1 -> MMPP/5(rn)
  Constant/1 -> MMPP/4(M)
  MMPP/1(x) -> X/1
  MMPP/4(t) -> Scope/1, t/1
  MMPP/2(T) -> T/1
  T/1 -> MMPP/2("T ")
  X/1 -> MMPP/1("x ")

== system QueuingSys/Distro/MMPPArrivalTime51 ==
  MMPPArrivalTime : TriggerPort  TriggerType=function-call  IsSimulinkFunction=on  FunctionName=MMPPArrivalTime51  VariantControl=Variant
  Constant : Constant  Value=[0.27477589633085 0.72522410366915;0.576167588252239 0.423832411747761]  SampleTime=-1
  D : Memory  InitialCondition=[0.679664293958122;0.0795688618013785]  InheritSampleTime=on
  MMPP : MATLAB Function  TreatAsAtomicUnit=on
  Scope : Scope
  Scope1 : Scope
  T : Memory  InitialCondition=[0 0.0601305715476238]  InheritSampleTime=on
  Uniform Random Number : UniformRandomNumber  Minimum=0  Seed=randi(5000)
  X : Memory  InitialCondition=1  InheritSampleTime=on
  t : ArgOut  DisableCoverage=on  ArgumentName=t
  wires:
  MMPP/5(lambda) -> Scope1/1
  D/1 -> MMPP/3("D ")
  MMPP/3(D) -> D/1
  Uniform Random Number/1 -> MMPP/5(rn)
  Constant/1 -> MMPP/4(M)
  MMPP/1(x) -> X/1
  MMPP/4(t) -> Scope/1, t/1
  MMPP/2(T) -> T/1
  T/1 -> MMPP/2("T ")
  X/1 -> MMPP/1("x ")

== system QueuingSys/Distro/MMPPArrivalTime52 ==
  MMPPArrivalTime : TriggerPort  TriggerType=function-call  IsSimulinkFunction=on  FunctionName=MMPPArrivalTime52  VariantControl=Variant
  Constant : Constant  Value=[0.0779456373812396 0.225274098754333 0.135235329503905 0.322160116791718 0.239384817568805;0.237603595831951 0.195901606332091 0.209668820848791 0.117585415067075 0.239240561920092;0.10094128161487 0.306255810576098 0.105545511079908 0.235267858982242 0.251989537746883;0.0317906697226869 0.0912138240831371 0.361158339860435 0.418438011318553 0.0973991550151886;0.344674187629098 0.328778261982713 0.177310589680979 0.0983342844648327 0.050902676242377]  SampleTime=-1
  D : Memory  InitialCondition=[0.980096005521268;0.751684027310974]  InheritSampleTime=on
  MMPP : MATLAB Function  TreatAsAtomicUnit=on
  Scope : Scope
  Scope1 : Scope
  T : Memory  InitialCondition=[0 1.32214312124926]  InheritSampleTime=on
  Uniform Random Number : UniformRandomNumber  Minimum=0  Seed=randi(5000)
  X : Memory  InitialCondition=5  InheritSampleTime=on
  t : ArgOut  DisableCoverage=on  ArgumentName=t
  wires:
  MMPP/5(lambda) -> Scope1/1
  D/1 -> MMPP/3("D ")
  MMPP/3(D) -> D/1
  Uniform Random Number/1 -> MMPP/5(rn)
  Constant/1 -> MMPP/4(M)
  MMPP/1(x) -> X/1
  MMPP/4(t) -> Scope/1, t/1
  MMPP/2(T) -> T/1
  T/1 -> MMPP/2("T ")
  X/1 -> MMPP/1("x ")

== system QueuingSys/Distro/MMPPArrivalTime53 ==
  MMPPArrivalTime : TriggerPort  TriggerType=function-call  IsSimulinkFunction=on  FunctionName=MMPPArrivalTime53  VariantControl=Variant
  Constant : Constant  Value=[0.123213782072751 0.0203564984206003 0.257051566111025 0.0145943311681688 0.0816876671703166 0.134023465595343 0.2585969637835 0.110475725678296;0.0177158527683463 0.194973002202457 0.12651531765153 0.114307978366439 0.0161070662064469 0.155504816989333 0.161669538323955 0.213206427491493;0.0344595627708055 0.124382621870903 0.173362716325991 0.0550418448821959 0.182709438022144 0.166633381790352 0.093981667089674 0.169428767247933;0.170175469423192 0.0369170999924753 0.013784091076386 0.147927274138185 0.0958134249132087 0.195744315289456 0.19364534372614 0.145992981440957;0.201811926034737 0.11150230943796 0.14620939075993 0.132613560755162 0.168392899815457 0.18383901638292 0.0311142203307919 0.024516676483042;0.185902766042658 0.153371383875054 0.0286654140386129 0.0177500774355355 0.266231807527502 0.0101540434889089 0.189511404901813 0.148413102689917;0.0941915976279465 0.113587544400254 0.11079634693523 0.162219066048839 0.158751736041027 0.164944426900267 0.107942998113772 0.0875662839326654;0.125359025190266 0.172346379619826 0.143719398120004 0.170339054795389 0.172131272820563 0.112197209524467 0.0917269017918102 0.0121807581376756]  SampleTime=-1
  D : Memory  InitialCondition=[0.805203215911553;0.786655637028361]  InheritSampleTime=on
  MMPP : MATLAB Function  TreatAsAtomicUnit=on
  Scope : Scope
  Scope1 : Scope
  T : Memory  InitialCondition=[0 1.31632258328505]  InheritSampleTime=on
  Uniform Random Number : UniformRandomNumber  Minimum=0  Seed=randi(5000)
  X : Memory  InitialCondition=4  InheritSampleTime=on
  t : ArgOut  DisableCoverage=on  ArgumentName=t
  wires:
  MMPP/5(lambda) -> Scope1/1
  D/1 -> MMPP/3("D ")
  MMPP/3(D) -> D/1
  Uniform Random Number/1 -> MMPP/5(rn)
  Constant/1 -> MMPP/4(M)
  MMPP/1(x) -> X/1
  MMPP/4(t) -> Scope/1, t/1
  MMPP/2(T) -> T/1
  T/1 -> MMPP/2("T ")
  X/1 -> MMPP/1("x ")

== system QueuingSys/Distro/MMPPArrivalTime54 ==
  MMPPArrivalTime : TriggerPort  TriggerType=function-call  IsSimulinkFunction=on  FunctionName=MMPPArrivalTime54  VariantControl=Variant
  Constant : Constant  Value=[0.0425375316354311 0.957462468364569;0.493384015353972 0.506615984646028]  SampleTime=-1
  D : Memory  InitialCondition=[0.48914740808751;0.284127022809931]  InheritSampleTime=on
  MMPP : MATLAB Function  TreatAsAtomicUnit=on
  Scope : Scope
  Scope1 : Scope
  T : Memory  InitialCondition=[0 0.320034256183147]  InheritSampleTime=on
  Uniform Random Number : UniformRandomNumber  Minimum=0  Seed=randi(5000)
  X : Memory  InitialCondition=1  InheritSampleTime=on
  t : ArgOut  DisableCoverage=on  ArgumentName=t
  wires:
  MMPP/5(lambda) -> Scope1/1
  D/1 -> MMPP/3("D ")
  MMPP/3(D) -> D/1
  Uniform Random Number/1 -> MMPP/5(rn)
  Constant/1 -> MMPP/4(M)
  MMPP/1(x) -> X/1
  MMPP/4(t) -> Scope/1, t/1
  MMPP/2(T) -> T/1
  T/1 -> MMPP/2("T ")
  X/1 -> MMPP/1("x ")

== system QueuingSys/Distro/MMPPArrivalTime55 ==
  MMPPArrivalTime : TriggerPort  TriggerType=function-call  IsSimulinkFunction=on  FunctionName=MMPPArrivalTime55  VariantControl=Variant
  Constant : Constant  Value=[0.322744310179396 0.161126721845851 0.516128967974753;0.393346289404341 0.250659781843798 0.35599392875186;0.360441015160688 0.329883638020048 0.309675346819264]  SampleTime=-1
  D : Memory  InitialCondition=[0.355807120256821;0.193194442421816]  InheritSampleTime=on
  MMPP : MATLAB Function  TreatAsAtomicUnit=on
  Scope : Scope
  Scope1 : Scope
  T : Memory  InitialCondition=[0 0.148193777445589]  InheritSampleTime=on
  Uniform Random Number : UniformRandomNumber  Minimum=0  Seed=randi(5000)
  X : Memory  InitialCondition=3  InheritSampleTime=on
  t : ArgOut  DisableCoverage=on  ArgumentName=t
  wires:
  MMPP/5(lambda) -> Scope1/1
  D/1 -> MMPP/3("D ")
  MMPP/3(D) -> D/1
  Uniform Random Number/1 -> MMPP/5(rn)
  Constant/1 -> MMPP/4(M)
  MMPP/1(x) -> X/1
  MMPP/4(t) -> Scope/1, t/1
  MMPP/2(T) -> T/1
  T/1 -> MMPP/2("T ")
  X/1 -> MMPP/1("x ")

== system QueuingSys/Distro/MMPPArrivalTime56 ==
  MMPPArrivalTime : TriggerPort  TriggerType=function-call  IsSimulinkFunction=on  FunctionName=MMPPArrivalTime56  VariantControl=Variant
  Constant : Constant  Value=[0.271279823615462 0.728720176384539;0.404893195333095 0.595106804666904]  SampleTime=-1
  D : Memory  InitialCondition=[0.789344549208544;0.350928314133683]  InheritSampleTime=on
  MMPP : MATLAB Function  TreatAsAtomicUnit=on
  Scope : Scope
  Scope1 : Scope
  T : Memory  InitialCondition=[0 0.174999743290798]  InheritSampleTime=on
  Uniform Random Number : UniformRandomNumber  Minimum=0  Seed=randi(5000)
  X : Memory  InitialCondition=2  InheritSampleTime=on
  t : ArgOut  DisableCoverage=on  ArgumentName=t
  wires:
  MMPP/5(lambda) -> Scope1/1
  D/1 -> MMPP/3("D ")
  MMPP/3(D) -> D/1
  Uniform Random Number/1 -> MMPP/5(rn)
  Constant/1 -> MMPP/4(M)
  MMPP/1(x) -> X/1
  MMPP/4(t) -> Scope/1, t/1
  MMPP/2(T) -> T/1
  T/1 -> MMPP/2("T ")
  X/1 -> MMPP/1("x ")
